simulink model "MRAC_quadrotor_attitude_control"  (R2017a)
settings: Solver=ode45  StartTime=0.0  StopTime=500  FixedStep=0.0001  RelTol=1e3  SampleTimeConstraint=STIndependent  EnableMultiTasking=on
undefined symbols (not defined in the file): DiscIntNeverNeededParam
libraries: dspmtrx3 x6, vrlib x2, neural x1, sharedutil x1
CloseFcn:
  | rtwprivate ssgencode ModelCloseRequest controller
settings Model: Creator=acer  LastModifiedBy=MAQ
settings SolverCC: ZeroCrossControl=DisableAll  AutoInsertRateTranBlk=on
settings DataIOCC: LimitDataPoints=on  SaveFormat=Array  SignalLoggingSaveFormat=ModelDataLogs
settings OptimizationCC: ExpressionDepthLimit=2147483647  LifeSpan=inf
settings DebuggingCC: SaveWithParameterizedLinksMsg=none  UnderspecifiedInitializationDetection=Classic  MergeDetectMultiDrivingBlocksExec=none  SolverPrmCheckMsg=warning  FcnCallInpInsideContextMsg=warning  StateNameClashWarn=warning  SFUnexpectedBacktrackingDiag=warning  SFNoUnconditionalDefaultTransitionDiag=warning  SFExecutionAtInitializationDiag=none
settings HardwareCC: ProdBitPerPointer=32  ProdBitPerSizeT=32  ProdBitPerPtrDiffT=32  ProdLargestAtomicFloat=None  ProdIntDivRoundTo=Undefined  ProdEndianess=Unspecified  ProdWordSize=32  ProdHWDeviceType=32-bit Generic
settings ModelReferenceCC: PropagateSignalLabelsOutOfModel=off
settings GRTTargetCC: TargetLangStandard=C89/C90 (ANSI)  GeneratePreprocessorConditionals=Disable all  CombineOutputUpdateFcns=off  GRTInterface=on
settings ConfigComp: CovMetricSettings=dw  CovHtmlReporting=on  CovSaveCumulativeToWorkspaceVar=on  CovSaveSingleToWorkspaceVar=on  CovExternalEMLEnable=off

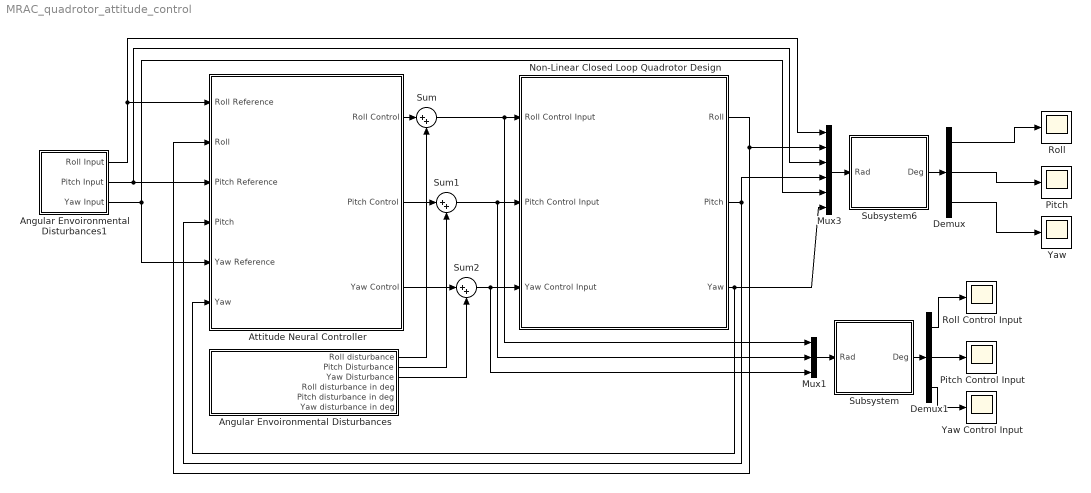
== system MRAC_quadrotor_attitude_control ==
  Angular Envoironmental Disturbances : Subsystem
  Angular Envoironmental Disturbances1 : Subsystem
  Attitude Neural Controller : Subsystem
  Demux : Demux  Outputs=[2,2,2]
  Demux1 : Demux  Outputs=3
  Mux1 : Mux  Inputs=3
  Mux3 : Mux  Inputs=6
  Non-Linear Closed Loop Quadrotor Design : Subsystem
  Pitch : Scope
  Pitch Control Input : Scope
  Roll : Scope
  Roll Control Input : Scope
  Subsystem : Subsystem
  Subsystem6 : Subsystem
  Sum : Sum  Inputs=|++
  Sum1 : Sum  Inputs=|++
  Sum2 : Sum  Inputs=|++
  Yaw : Scope
  Yaw Control Input : Scope
  wires:
  Non-Linear Closed Loop Quadrotor Design/1(Roll) -> Mux3/2, Attitude Neural Controller/2(Roll)
  Angular Envoironmental Disturbances1/1(Roll Input) -> Attitude Neural Controller/1(Roll Reference), Mux3/1
  Demux1/1 -> Roll Control Input/1
  Angular Envoironmental Disturbances1/2(Pitch Input) -> Mux3/3, Attitude Neural Controller/3(Pitch Reference)
  Non-Linear Closed Loop Quadrotor Design/2(Pitch) -> Attitude Neural Controller/4(Pitch), Mux3/4
  Demux1/2 -> Pitch Control Input/1
  Sum1/1 -> Mux1/2, Non-Linear Closed Loop Quadrotor Design/2(Pitch Control Input)
  Sum/1 -> Mux1/1, Non-Linear Closed Loop Quadrotor Design/1(Roll Control Input)
  Sum2/1 -> Mux1/3, Non-Linear Closed Loop Quadrotor Design/3(Yaw Control Input)
  Non-Linear Closed Loop Quadrotor Design/3(Yaw) -> Attitude Neural Controller/6(Yaw), Mux3/6
  Angular Envoironmental Disturbances1/3(Yaw Input) -> Attitude Neural Controller/5(Yaw Reference), Mux3/5
  Demux1/3 -> Yaw Control Input/1
  Mux3/1 -> Subsystem6/1(Rad)
  Subsystem6/1(Deg) -> Demux/1
  Demux/2 -> Pitch/1
  Mux1/1 -> Subsystem/1(Rad)
  Subsystem/1(Deg) -> Demux1/1
  Attitude Neural Controller/3(Yaw Control) -> Sum2/1
  Angular Envoironmental Disturbances/3(Yaw Disturbance) -> Sum2/2
  Attitude Neural Controller/2(Pitch Control) -> Sum1/1
  Angular Envoironmental Disturbances/2(Pitch Disturbance) -> Sum1/2
  Attitude Neural Controller/1(Roll Control) -> Sum/1
  Angular Envoironmental Disturbances/1(Roll disturbance) -> Sum/2
  Demux/1 -> Roll/1
  Demux/3 -> Yaw/1

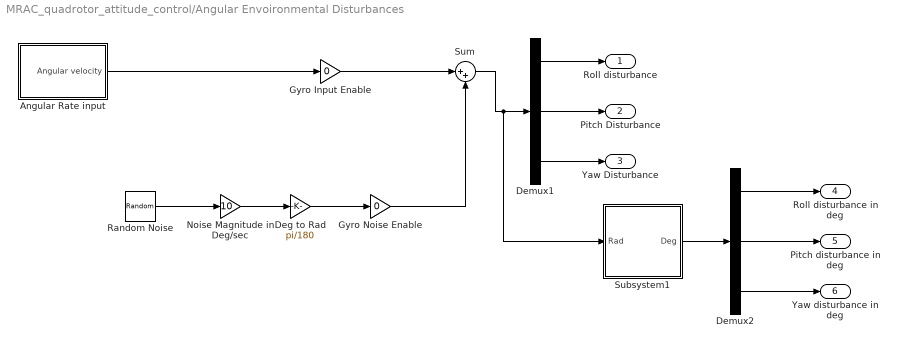
== system MRAC_quadrotor_attitude_control/Angular Envoironmental Disturbances ==
  Angular Rate input : Subsystem
  Deg to Rad : Gain  Gain=pi/180
  Demux1 : Demux  Outputs=3
  Demux2 : Demux  Outputs=3
  Gyro Input Enable : Gain  Gain=0
  Gyro Noise Enable : Gain  Gain=0
  Noise Magnitude in Deg/sec : Gain  Gain=10
  Random Noise : RandomNumber  Variance=0.25  SampleTime=0
  Subsystem1 : Subsystem
  Sum : Sum  Inputs=|++
  Roll disturbance : Outport
  Pitch Disturbance : Outport  Port=2
  Yaw Disturbance : Outport  Port=3
  Roll disturbance in deg : Outport  Port=4
  Pitch disturbance in deg : Outport  Port=5
  Yaw disturbance in deg : Outport  Port=6
  wires:
  Random Noise/1 -> Noise Magnitude in Deg/sec/1
  Sum/1 -> Subsystem1/1(Rad), Demux1/1
  Gyro Noise Enable/1 -> Sum/2
  Angular Rate input/1(Angular velocity) -> Gyro Input Enable/1
  Deg to Rad/1 -> Gyro Noise Enable/1
  Noise Magnitude in Deg/sec/1 -> Deg to Rad/1
  Gyro Input Enable/1 -> Sum/1
  Demux1/1 -> Roll disturbance/1
  Demux1/2 -> Pitch Disturbance/1
  Demux1/3 -> Yaw Disturbance/1
  Subsystem1/1(Deg) -> Demux2/1
  Demux2/1 -> Roll disturbance in deg/1
  Demux2/3 -> Yaw disturbance in deg/1
  Demux2/2 -> Pitch disturbance in deg/1

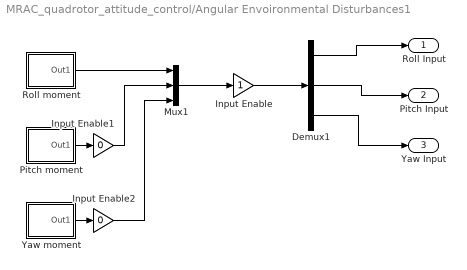
== system MRAC_quadrotor_attitude_control/Angular Envoironmental Disturbances1 ==
  Demux1 : Demux  Outputs=3
  Input Enable : Gain
  Input Enable1 : Gain  Gain=0
  Input Enable2 : Gain  Gain=0
  Mux1 : Mux  Inputs=3
  Pitch moment : Subsystem  mask(timed input){t=[0 100 100 500], u=[0 0 25 25]*pi/180}
      mask prompts: t "time values:"; u "input values"
      mask Display: plot(t,u)
  Roll moment : Subsystem  mask(timed input){t=[0 200 200 500], u=[0 0 20 20]*pi/180}
      mask prompts: t "time values:"; u "input values"
      mask Display: plot(t,u)
  Yaw moment : Subsystem  mask(timed input){t=[0 300 300 500], u=[0 0 10 10]*pi/180}
      mask prompts: t "time values:"; u "input values"
      mask Display: plot(t,u)
  Roll Input : Outport
  Pitch Input : Outport  Port=2
  Yaw Input : Outport  Port=3
  wires:
  Roll moment/1(Out1) -> Mux1/1
  Pitch moment/1(Out1) -> Input Enable1/1
  Yaw moment/1(Out1) -> Input Enable2/1
  Demux1/1 -> Roll Input/1
  Demux1/2 -> Pitch Input/1
  Demux1/3 -> Yaw Input/1
  Input Enable/1 -> Demux1/1
  Mux1/1 -> Input Enable/1
  Input Enable1/1 -> Mux1/2
  Input Enable2/1 -> Mux1/3

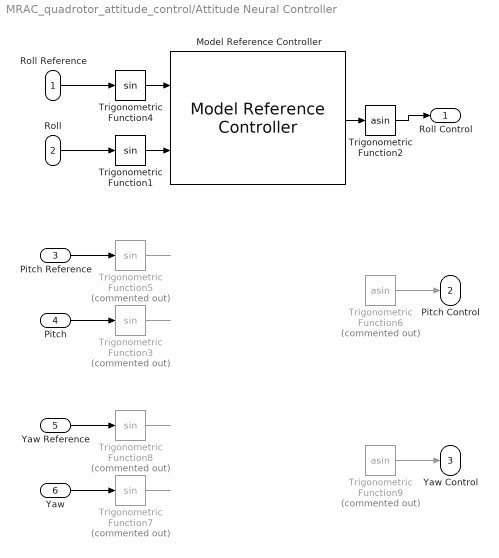
== system MRAC_quadrotor_attitude_control/Attitude Neural Controller ==
  Roll Reference : Inport
  Roll : Inport  Port=2
  Pitch Reference : Inport  Port=3
  Pitch : Inport  Port=4
  Yaw Reference : Inport  Port=5
  Yaw : Inport  Port=6
  Model Reference Controller : neural/Control Systems/Model Reference Controller  Nrc=4  Nic=3  Njc=4  IW_y=[-0.26400634085531088 0.11362328074890946 0.76949015312332025 1.005941348454747;0.36688412438777618 -0.0065967410290466979 -0.72033985218232333 -0.88912388699089739;-0.50358139131277091 0.77939865285332366 0.45366564233329087 0.20305295002900911;0.69691551574309296 0.93834213965429825 0.99228413522118419 0.46539351004482765;-0.59091694955932106 0.27420026736245862 -0.55638905843394881 -0.1844617097356944;-1.1767358237096723 -0.42345585278014547 -1.376668685165205 -1.9008307651836231;0.91466033120602253 -0.41297814120526233 -0.26385222896894323 0.77394756493515449;0.29502607955624394 -0.52311745453581648 -0.39832939881783536 0.37380188688815252;1.0660136206391706 0.91244449330040633 0.99696460523911079 0.49155115383902304;0.63070297319256308 -0.38669531637003984 0.59581348825373337 -0.21032775941831702]  IW_u=[0.56042977945772532 1.0486777442660933 2.1987425118943289;-1.6889164657557667 -0.80321266338753694 -0.9192800619649194;-1.8541863287530997 -0.20017097188284924 -0.60708641279665343;-0.28001378328225929 -1.1150075654652816 1.0207940783869573;-0.70499564957587701 -0.95237632324574006 0.23088874925544114;-0.42189625740733028 -2.3705195154705936 -4.0674084796699121;0.7474100462947203 -1.1953524768000803 -1.3655327562504367;1.3761003380140078 -1.3942056469524908 -0.91047566712262429;1.2032143316328423 1.5376001733686817 0.34323566602274552;-1.1228995990140889 -0.57599779319136679 -1.5199715167734213]  IW_r=[0.13929880088084767 -0.71123019484301042 -0.25515608640194143 -0.041422524854309049;0.13611795317236861 0.019832696517312072 0.70934291910829628 -0.39652942402808944;0.33631471976119631 -0.52824952533632286 -0.60220437280042194 -0.505246106197206;0.30881393403028395 -0.14255401474162388 -0.66488436571113796 0.33691864529663251;0.40040038631379271 1.0480728407462128 0.55697999347242622 -0.030184834439182788;0.90955877692360643 0.95199087143149452 1.0833619369597556 0.34265164308091162;0.67014617449781022 0.61015340408200858 0.74157586751999494 -0.30252864375186672;-0.72603142613625271 -0.12043858389185157 1.0571323958095122 0.37622613209432421;-0.39254518098273627 -1.1001741292886296 0.29052193957884587 -0.33761877898832748;-1.1572293229757462 -0.018972447365077257 -0.29945439714169159 -0.95018887104406002]  B1_c=[0.64282150723717402;-1.0714314143688932;0.15436795978763335;0.73690626046510621;-0.074033003191508698;0.40729244123106328;0.22841516922084279;0.61431964891831858;0.14949779394883281;1.7263533850660762]  B2_c=0.31484879587640524  LW_c=[0.036083219740493624 -0.017033421322474054 -0.44456589280132919 0.06417024420824434 0.59729580944885596 -0.040970357809656605 0.63106519715641407 -0.78172709286945619 -0.16468842249372001 0.060969010733739011]  retraining_c=25  max_i_int=0  min_i_int=0  max_r_int=400  min_r_int=100  Ts=0.05  S1=5  Ni=2  Nj=2  sim_file=0  trainfun=trainlm  Use_validation=0  Use_Testing=1  Use_Inc_training=0  Use_previous_weights=1  max_i=1  min_i=-1  max_r=1  min_r=-1  sam_training=0  sam_training_c=5000  epochs=200  epochs_c=30  minp=-0.93969262078590832  maxp=0.93969262078590832  mint=-0.9848038138280788  maxt=0.93969262078590832  Normalize=0  IW=[-0.025013062042015918 0.004136464686980838;-0.97797176081375736 -0.695916466928859;-0.039432618863616486 -0.0038877108883655742;-0.98427976015700624 -0.48483062015731698;-0.001724540600165126 0.0020387649276496118]  LW1_2=[1.8522611518720808 -0.80388200875864657;-1.5185066206607776 0.20172978663592384;0.40524480460798651 -1.2719330598899341;-1.1018603734955705 1.432108945243316;-1.176149127779192 0.62707492245559471]  LW2_1=[0.62787707146920846 0.0018729990102923592 -0.47303644161933917 0.004122445633035327 -1.6196132281773281]  B1=[-1.7854455549452175;0.68675602723942142;0.43375087295602627;-0.21370894191486062;-0.66468364827367854]  B2=-0.15531704723775702  S1c=10  Limit_output=0  min_output=0  max_output=0  Ref_file=0
      settings: SourceProductName=Neural Network Toolbox  SourceProductBaseCode=NN
  Trigonometric Function1 : Trigonometry
  Trigonometric Function2 : Trigonometry  Operator=asin  OutputSignalType=real
  Trigonometric Function{3,5,7..8} (4 alike) : Trigonometry  Commented=on
  Trigonometric Function4 : Trigonometry
  Trigonometric Function6 : Trigonometry  Commented=on  Operator=asin  OutputSignalType=real
  Trigonometric Function9 : Trigonometry  Commented=on  Operator=asin  OutputSignalType=real
  Roll Control : Outport
  Pitch Control : Outport  Port=2
  Yaw Control : Outport  Port=3
  wires:
  Trigonometric Function5/1 -> ?
  Model Reference Controller/1 -> Trigonometric Function2/1
  Trigonometric Function1/1 -> Model Reference Controller/2
  Trigonometric Function4/1 -> Model Reference Controller/1
  Trigonometric Function3/1 -> ?
  Trigonometric Function6/1 -> Pitch Control/1
  Trigonometric Function2/1 -> Roll Control/1
  ? -> Trigonometric Function6/1
  Pitch/1 -> Trigonometric Function3/1
  Pitch Reference/1 -> Trigonometric Function5/1
  Roll Reference/1 -> Trigonometric Function4/1
  Roll/1 -> Trigonometric Function1/1
  Yaw/1 -> Trigonometric Function7/1
  Yaw Reference/1 -> Trigonometric Function8/1
  ? -> Trigonometric Function9/1
  Trigonometric Function7/1 -> ?
  Trigonometric Function8/1 -> ?
  Trigonometric Function9/1 -> Yaw Control/1

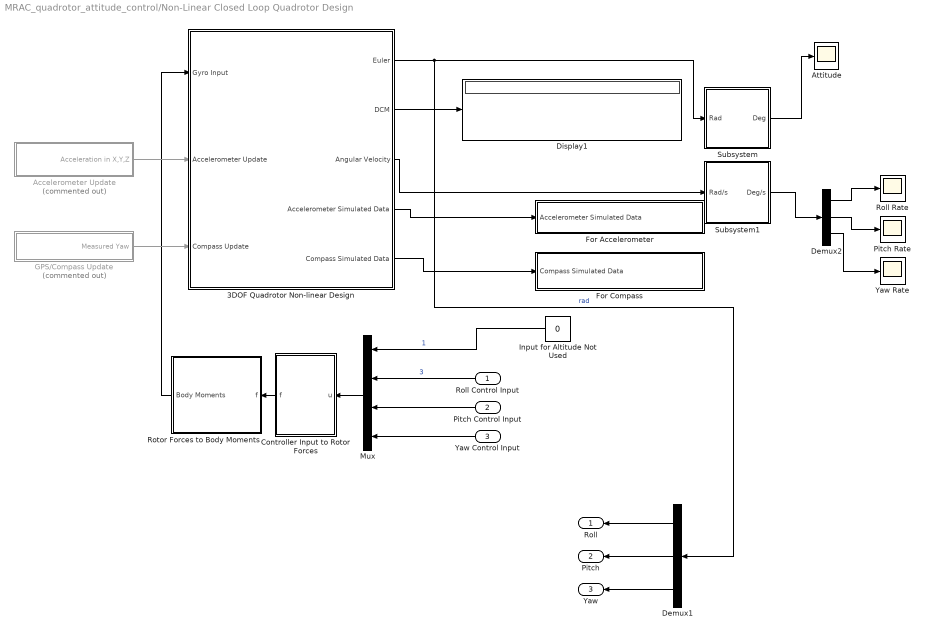
== system MRAC_quadrotor_attitude_control/Non-Linear Closed Loop Quadrotor Design ==
  Roll Control Input : Inport
  Pitch Control Input : Inport  Port=2
  Yaw Control Input : Inport  Port=3
  3DOF Quadrotor Non-linear Design : Subsystem
  Accelerometer Update : Subsystem  Commented=on
  Attitude : Scope
  Controller Input to Rotor Forces : Subsystem
  Demux1 : Demux  Outputs=3
  Demux2 : Demux  Outputs=3
  Display1 : Display
  For Accelerometer : Subsystem
  For Compass : Subsystem
  GPS/Compass Update : Subsystem  Commented=on
  Input for Altitude Not Used : Constant  Value=0
  Mux : Mux
  Pitch Rate : Scope
  Roll Rate : Scope
  Rotor Forces to Body Moments : Subsystem
  Subsystem : Subsystem
  Subsystem1 : Subsystem
  Yaw Rate : Scope
  Roll : Outport
  Pitch : Outport  Port=2
  Yaw : Outport  Port=3
  wires:
  Controller Input to Rotor Forces/1(f) -> Rotor Forces to Body Moments/1(f)
  3DOF Quadrotor Non-linear Design/1(Euler) -> Demux1/1, Subsystem/1(Rad)  "rad"
  Rotor Forces to Body Moments/1(Body Moments) -> 3DOF Quadrotor Non-linear Design/1(Gyro Input)
  Accelerometer Update/1(Acceleration in X,Y,Z) -> 3DOF Quadrotor Non-linear Design/2(Accelerometer Update)
  GPS/Compass Update/1(Measured Yaw) -> 3DOF Quadrotor Non-linear Design/3(Compass Update)
  3DOF Quadrotor Non-linear Design/2(DCM) -> Display1/1
  Subsystem/1(Deg) -> Attitude/1
  Subsystem1/1(Deg/s) -> Demux2/1
  Demux2/1 -> Roll Rate/1
  Demux2/2 -> Pitch Rate/1
  Demux2/3 -> Yaw Rate/1
  3DOF Quadrotor Non-linear Design/3("Angular Velocity ") -> Subsystem1/1(Rad/s)
  3DOF Quadrotor Non-linear Design/4(Accelerometer Simulated Data) -> For Accelerometer/1(Accelerometer Simulated Data)
  3DOF Quadrotor Non-linear Design/5(Compass Simulated Data) -> For Compass/1(Compass Simulated Data)
  Input for Altitude Not Used/1 -> Mux/1  "1"
  Roll Control Input/1 -> Mux/2  "3"
  Mux/1 -> Controller Input to Rotor Forces/1(u)
  Demux1/1 -> Roll/1
  Pitch Control Input/1 -> Mux/3
  Demux1/2 -> Pitch/1
  Yaw Control Input/1 -> Mux/4
  Demux1/3 -> Yaw/1

== system MRAC_quadrotor_attitude_control/Subsystem ==
  Rad : Inport
  Constant : Constant  Value=180/pi
  Product1 : Product  RndMeth=Zero
  Deg : Outport
  wires:
  Constant/1 -> Product1/2
  Rad/1 -> Product1/1
  Product1/1 -> Deg/1

== system MRAC_quadrotor_attitude_control/Subsystem6 ==
  Rad : Inport
  Constant : Constant  Value=180/pi
  Product1 : Product  RndMeth=Zero
  Deg : Outport
  wires:
  Constant/1 -> Product1/2
  Rad/1 -> Product1/1
  Product1/1 -> Deg/1

== system MRAC_quadrotor_attitude_control/Angular Envoironmental Disturbances/Angular Rate input ==
  Mux : Mux  Inputs=3
  Pitch moment : Subsystem  mask(timed input){t=[0 100 100 200 200 300 300 400 400 500], u=[0 0 50 50 0 0 -50 -50 0 0]*pi/180*0}
      mask prompts: t "time values:"; u "input values"
      mask Display: plot(t,u)
  Roll moment : Subsystem  mask(timed input){t=[0 100 100 200 200 300 300 400 400 500], u=[0 0 50 50 0 0 -50 -50 0 0]*pi/180}
      mask prompts: t "time values:"; u "input values"
      mask Display: plot(t,u)
  Yaw moment : Subsystem  mask(timed input){t=[0 200 200 300 300 400 400 500], u=[0 0 45 45 0 0 -45 -45]*pi/180*0}
      mask prompts: t "time values:"; u "input values"
      mask Display: plot(t,u)
  Angular velocity : Outport
  wires:
  Roll moment/1(Out1) -> Mux/1
  Pitch moment/1(Out1) -> Mux/2
  Yaw moment/1(Out1) -> Mux/3
  Mux/1 -> Angular velocity/1

== system MRAC_quadrotor_attitude_control/Angular Envoironmental Disturbances/Subsystem1 ==
  Rad : Inport
  Constant : Constant  Value=180/pi
  Product1 : Product  RndMeth=Zero
  Deg : Outport
  wires:
  Constant/1 -> Product1/2
  Rad/1 -> Product1/1
  Product1/1 -> Deg/1

== system MRAC_quadrotor_attitude_control/Angular Envoironmental Disturbances1/Pitch moment ==
  From Workspace : FromWorkspace  VariableName=[t',u']  SampleTime=0
  Out1 : Outport
  wires:
  From Workspace/1 -> Out1/1

== system MRAC_quadrotor_attitude_control/Angular Envoironmental Disturbances1/Roll moment ==
  From Workspace : FromWorkspace  VariableName=[t',u']  SampleTime=0
  Out1 : Outport
  wires:
  From Workspace/1 -> Out1/1

== system MRAC_quadrotor_attitude_control/Angular Envoironmental Disturbances1/Yaw moment ==
  From Workspace : FromWorkspace  VariableName=[t',u']  SampleTime=0
  Out1 : Outport
  wires:
  From Workspace/1 -> Out1/1

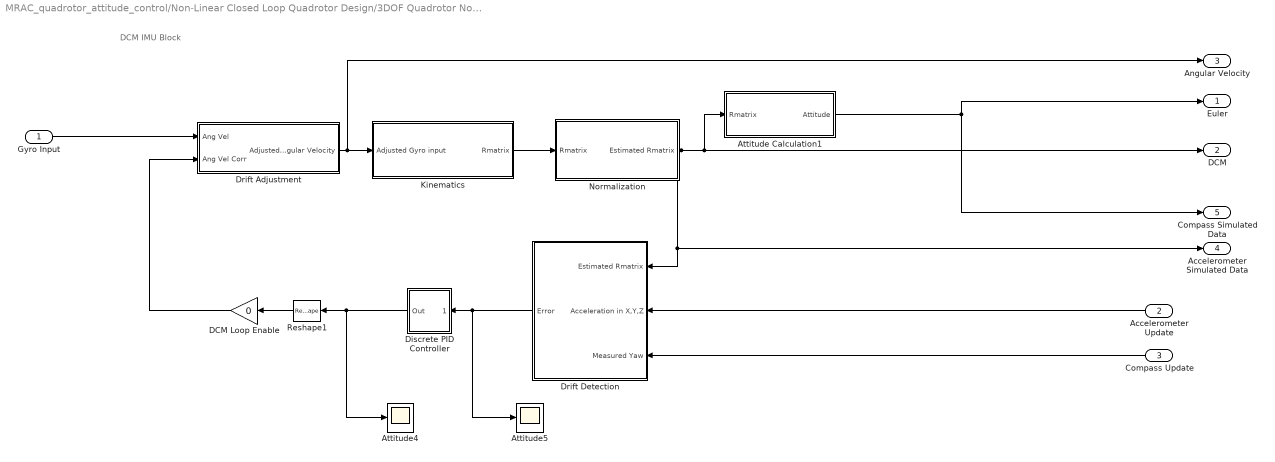
== system MRAC_quadrotor_attitude_control/Non-Linear Closed Loop Quadrotor Design/3DOF Quadrotor Non-linear Design ==
  note: DCM IMU Block
  Gyro Input : Inport
  Accelerometer Update : Inport  Port=2
  Compass Update : Inport  Port=3
  Attitude Calculation1 : Subsystem
  Attitude4 : Scope
  Attitude5 : Scope
  DCM Loop Enable : Gain  Gain=0
  Discrete PID Controller : Subsystem  AncestorBlock=|  DialogController=POWERSYS.PowerSysDialog  mask(Discrete PID Controller){Kp=5, Ki=2, Kd=0, TcD=0, Par_Limits=[1e6 -1e6], Init=0, Ts=1}
      | powerlib_extras/Discrete 
      | Control Blocks/Discrete
      | PID Controller
      mask prompts: Kp "Proportional gain (Kp):"; Ki "Integral gain (Ki):"; Kd "Derivative gain (Kd):"; TcD "Time constant for derivative (s):"; Par_Limits "Output limits: [ Upper   Lower ]"; Init "Output initial value:"; Ts "Sample time:"
      mask help: This block implements a discrete PID controller.
      mask init:
      | UpperLimit=Par_Limits(1);
      | LowerLimit=Par_Limits(2);
      | power_initmask();
      mask Help: This block is part of a subset of blocks in the Extras library that does not have documentation associated with it, other than the block mask description.
      mask Display: disp('PID');
  Drift Adjustment : Subsystem
  Drift Detection : Subsystem
  Kinematics : Subsystem
  Normalization : Subsystem
  Reshape1 : Reshape  OutputDimensionality=Column vector (2-D)
  Euler : Outport
  DCM : Outport  Port=2
  "Angular Velocity " : Outport  Port=3
  Accelerometer Simulated Data : Outport  Port=4
  Compass Simulated Data : Outport  Port=5
  wires:
  Attitude Calculation1/1(Attitude) -> Euler/1, Compass Simulated Data/1
  Drift Adjustment/1(Adjusted Angular Velocity) -> "Angular Velocity "/1, Kinematics/1(Adjusted Gyro input)
  Gyro Input/1 -> Drift Adjustment/1(Ang Vel)
  Compass Update/1 -> Drift Detection/3(Measured Yaw)
  Drift Detection/1(Error) -> Attitude5/1, Discrete PID Controller/1(Error)
  Discrete PID Controller/1(Out) -> Attitude4/1, Reshape1/1
  Accelerometer Update/1 -> Drift Detection/2(Acceleration in X,Y,Z)
  Reshape1/1 -> DCM Loop Enable/1
  DCM Loop Enable/1 -> Drift Adjustment/2(Ang Vel Corr)
  Normalization/1(Estimated Rmatrix) -> Accelerometer Simulated Data/1, Drift Detection/1(Estimated Rmatrix), Attitude Calculation1/1(Rmatrix), DCM/1
  Kinematics/1(Rmatrix) -> Normalization/1(Rmatrix)

== system MRAC_quadrotor_attitude_control/Non-Linear Closed Loop Quadrotor Design/Accelerometer Update ==
  Attitude2 : Scope
  From File : FromFile  FileName=acceleration_from_simulink  SampleTime=0
  Acceleration in X,Y,Z : Outport
  wires:
  From File/1 -> Attitude2/1, Acceleration in X,Y,Z/1

== system MRAC_quadrotor_attitude_control/Non-Linear Closed Loop Quadrotor Design/Controller Input to Rotor Forces ==
  u : Inport
  Matrix Multiply : Product  Multiplication=Matrix(*)
  inv(plant_model) : Constant  Value=|  VectorParams1D=off
      | [  -0.2500         0   -0.5000   -0.2500
      |  ;  -0.2500   -0.5000         0    0.2500
      |   ; -0.2500         0    0.5000   -0.2500
      |   ; -0.2500    0.5000         0    0.2500
      | ]
  f : Outport
  wires:
  inv(plant_model)/1 -> Matrix Multiply/1
  Matrix Multiply/1 -> f/1
  u/1 -> Matrix Multiply/2

== system MRAC_quadrotor_attitude_control/Non-Linear Closed Loop Quadrotor Design/For Accelerometer ==
  Accelerometer Simulated Data : Inport
  Embedded MATLAB Function1 : MATLAB Function  TreatAsAtomicUnit=on
  For acceleration : ToFile  Filename=acceleration_from_simulink.mat
  Mux : Mux  Inputs=3
  wires:
  Embedded MATLAB Function1/1(accel_x) -> Mux/1
  Embedded MATLAB Function1/3(accel_z) -> Mux/3
  Mux/1 -> For acceleration/1
  Embedded MATLAB Function1/2(accel_y) -> Mux/2
  Accelerometer Simulated Data/1 -> Embedded MATLAB Function1/1(R_t_n)

== system MRAC_quadrotor_attitude_control/Non-Linear Closed Loop Quadrotor Design/For Compass ==
  Compass Simulated Data : Inport
  Demux1 : Demux  Outputs=3
  For Compass : ToFile  Filename=yaw_from_simulink
  Terminator1 : Terminator
  Terminator2 : Terminator
  wires:
  Compass Simulated Data/1 -> Demux1/1
  Demux1/2 -> Terminator2/1
  Demux1/1 -> Terminator1/1
  Demux1/3 -> For Compass/1

== system MRAC_quadrotor_attitude_control/Non-Linear Closed Loop Quadrotor Design/GPS//Compass Update ==
  Attitude3 : Scope
  GPS/Compass Update : FromFile  FileName=yaw_from_simulink  SampleTime=0
  Subsystem2 : Subsystem
  Measured Yaw : Outport
  wires:
  GPS/Compass Update/1 -> Subsystem2/1(Rad), Measured Yaw/1
  Subsystem2/1(Deg) -> Attitude3/1

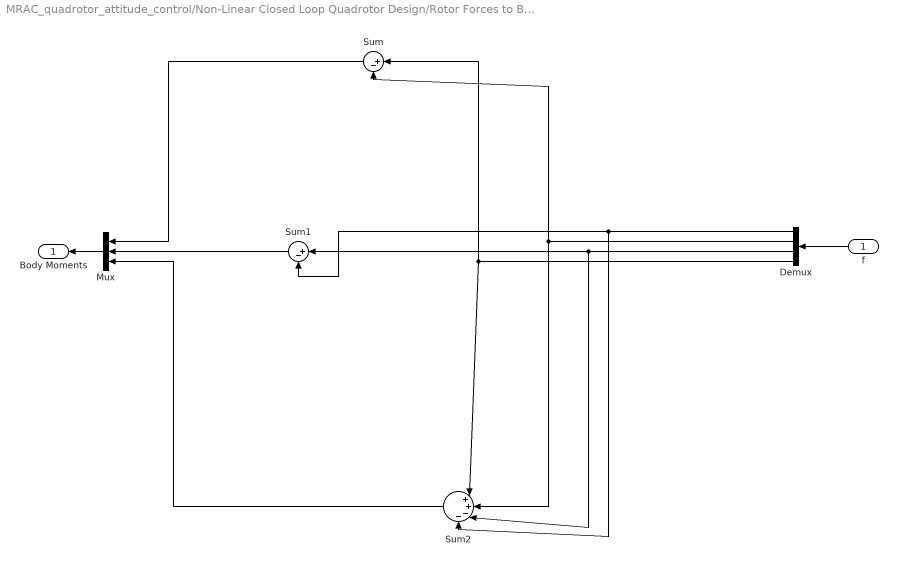
== system MRAC_quadrotor_attitude_control/Non-Linear Closed Loop Quadrotor Design/Rotor Forces to Body Moments ==
  f : Inport
  Demux : Demux
  Mux : Mux  Inputs=3
  Sum : Sum  Inputs=|+-
  Sum1 : Sum  Inputs=|+-
  Sum2 : Sum  Inputs=|++--
  Body Moments : Outport
  wires:
  Sum/1 -> Mux/1
  Sum1/1 -> Mux/2
  Sum2/1 -> Mux/3
  f/1 -> Demux/1
  Mux/1 -> Body Moments/1
  Demux/1 -> Sum1/2, Sum2/4
  Demux/2 -> Sum2/2, Sum/2
  Demux/3 -> Sum1/1, Sum2/3
  Demux/4 -> Sum2/1, Sum/1

== system MRAC_quadrotor_attitude_control/Non-Linear Closed Loop Quadrotor Design/Subsystem ==
  Rad : Inport
  Constant : Constant  Value=180/pi
  Product1 : Product  RndMeth=Zero
  Deg : Outport
  wires:
  Constant/1 -> Product1/2
  Rad/1 -> Product1/1
  Product1/1 -> Deg/1

== system MRAC_quadrotor_attitude_control/Non-Linear Closed Loop Quadrotor Design/Subsystem1 ==
  Rad/s : Inport
  Constant : Constant  Value=180/pi
  Product1 : Product  RndMeth=Zero
  Deg/s : Outport
  wires:
  Constant/1 -> Product1/2
  Rad/s/1 -> Product1/1
  Product1/1 -> Deg/s/1

== system MRAC_quadrotor_attitude_control/Angular Envoironmental Disturbances/Angular Rate input/Pitch moment ==
  From Workspace : FromWorkspace  VariableName=[t',u']  SampleTime=0
  Out1 : Outport
  wires:
  From Workspace/1 -> Out1/1

== system MRAC_quadrotor_attitude_control/Angular Envoironmental Disturbances/Angular Rate input/Roll moment ==
  From Workspace : FromWorkspace  VariableName=[t',u']  SampleTime=0
  Out1 : Outport
  wires:
  From Workspace/1 -> Out1/1

== system MRAC_quadrotor_attitude_control/Angular Envoironmental Disturbances/Angular Rate input/Yaw moment ==
  From Workspace : FromWorkspace  VariableName=[t',u']  SampleTime=0
  Out1 : Outport
  wires:
  From Workspace/1 -> Out1/1

== system MRAC_quadrotor_attitude_control/Non-Linear Closed Loop Quadrotor Design/3DOF Quadrotor Non-linear Design/Attitude Calculation1 ==
  Rmatrix : Inport
  Embedded MATLAB Function1 : MATLAB Function  TreatAsAtomicUnit=on
  Mux : Mux  Inputs=3
  Attitude : Outport
  wires:
  Embedded MATLAB Function1/1(Roll) -> Mux/1
  Mux/1 -> Attitude/1
  Rmatrix/1 -> Embedded MATLAB Function1/1(R_mat)
  Embedded MATLAB Function1/2(Pitch) -> Mux/2
  Embedded MATLAB Function1/3(Yaw) -> Mux/3

== system MRAC_quadrotor_attitude_control/Non-Linear Closed Loop Quadrotor Design/3DOF Quadrotor Non-linear Design/Discrete PID Controller ==
  note: Pierre Giroux, Gilbert Sybille
      | Power System Simulation Laboratory
      | IREQ, Hydro-Quebc
  note: Discrete PID Controller
  Error : Inport
  Discrete-Time Integrator : DiscreteIntegrator  InitialCondition=Init  SampleTime=Ts  LimitOutput=on  UpperSaturationLimit=UpperLimit  LowerSaturationLimit=LowerLimit  ICPrevOutput=DiscIntNeverNeededParam  ICPrevScaledInput=DiscIntNeverNeededParam
  Kp4 : Gain  Gain=Kp  SaturateOnIntegerOverflow=on  OutDataTypeStr=Inherit: Same as input  ParamDataTypeStr=Inherit: Same as input
  Kp5 : Gain  Gain=Ki  SaturateOnIntegerOverflow=on  OutDataTypeStr=Inherit: Same as input  ParamDataTypeStr=Inherit: Same as input
  Saturation2 : Saturate  UpperLimit=UpperLimit  LowerLimit=LowerLimit
  Sum6 : Sum  SaturateOnIntegerOverflow=on  InputSameDT=on  OutDataTypeStr=Inherit: Same as first input
  Out : Outport  InitialOutput=0
  wires:
  Error/1 -> Kp4/1, Kp5/1
  Sum6/1 -> Saturation2/1
  Kp5/1 -> Discrete-Time Integrator/1
  Kp4/1 -> Sum6/1
  Discrete-Time Integrator/1 -> Sum6/2
  Saturation2/1 -> Out/1

== system MRAC_quadrotor_attitude_control/Non-Linear Closed Loop Quadrotor Design/3DOF Quadrotor Non-linear Design/Drift Adjustment ==
  Ang Vel : Inport
  Ang Vel Corr : Inport  Port=2
  Sum : Sum  Inputs=|+-
  Adjusted Angular Velocity : Outport
  wires:
  Ang Vel/1 -> Sum/1
  Sum/1 -> Adjusted Angular Velocity/1
  Ang Vel Corr/1 -> Sum/2

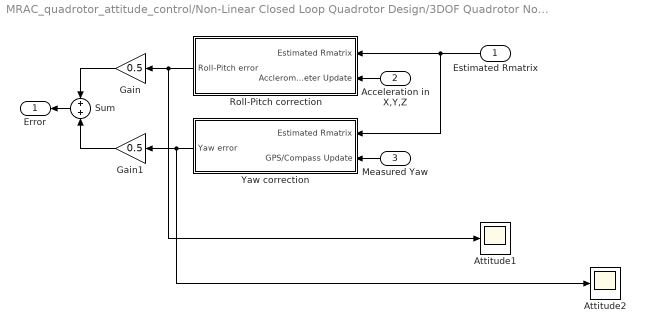
== system MRAC_quadrotor_attitude_control/Non-Linear Closed Loop Quadrotor Design/3DOF Quadrotor Non-linear Design/Drift Detection ==
  Estimated Rmatrix : Inport
  Acceleration in X,Y,Z : Inport  Port=2
  Measured Yaw : Inport  Port=3
  Attitude1 : Scope
  Attitude2 : Scope
  Gain : Gain  Gain=0.5
  Gain1 : Gain  Gain=0.5
  Roll-Pitch correction : Subsystem
  Sum : Sum
  Yaw correction : Subsystem
  Error : Outport
  wires:
  Roll-Pitch correction/1(Roll-Pitch error) -> Attitude1/1, Gain/1
  Yaw correction/1(Yaw error) -> Attitude2/1, Gain1/1
  Estimated Rmatrix/1 -> Roll-Pitch correction/1(Estimated Rmatrix), Yaw correction/1(Estimated Rmatrix)
  Acceleration in X,Y,Z/1 -> Roll-Pitch correction/2(Acclerometer Update)
  Measured Yaw/1 -> Yaw correction/2(GPS/Compass Update)
  Sum/1 -> Error/1
  Gain/1 -> Sum/1
  Gain1/1 -> Sum/2

== system MRAC_quadrotor_attitude_control/Non-Linear Closed Loop Quadrotor Design/3DOF Quadrotor Non-linear Design/Kinematics ==
  Adjusted Gyro input : Inport
  Demux : Demux  Outputs=3
  Embedded MATLAB Function : MATLAB Function  TreatAsAtomicUnit=on
  Memory : Memory
  Rmatrix : Outport
  wires:
  Demux/1 -> Embedded MATLAB Function/1(R_rate)
  Demux/2 -> Embedded MATLAB Function/2(P_rate)
  Demux/3 -> Embedded MATLAB Function/3(Y_rate)
  Embedded MATLAB Function/1(R_t) -> Memory/1, Rmatrix/1
  Memory/1 -> Embedded MATLAB Function/4(R_t_i)
  Adjusted Gyro input/1 -> Demux/1

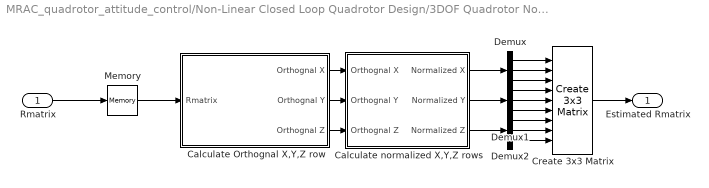
== system MRAC_quadrotor_attitude_control/Non-Linear Closed Loop Quadrotor Design/3DOF Quadrotor Non-linear Design/Normalization ==
  Rmatrix : Inport
  Calculate Orthognal X,Y,Z row : Subsystem
  Calculate normalized X,Y,Z rows : Subsystem
  Create 3x3 Matrix : sharedutil/Create 3x3 Matrix
  Demux : Demux  Outputs=3
  Demux1 : Demux  Outputs=3
  Demux2 : Demux  Outputs=3
  Memory : Memory
  Estimated Rmatrix : Outport
  wires:
  Calculate normalized X,Y,Z rows/1(Normalized X) -> Demux/1
  Calculate normalized X,Y,Z rows/2(Normalized Y) -> Demux1/1
  Calculate normalized X,Y,Z rows/3(Normalized Z) -> Demux2/1
  Demux/1 -> Create 3x3 Matrix/1
  Demux/2 -> Create 3x3 Matrix/2
  Demux/3 -> Create 3x3 Matrix/3
  Demux1/1 -> Create 3x3 Matrix/4
  Demux1/2 -> Create 3x3 Matrix/5
  Demux1/3 -> Create 3x3 Matrix/6
  Demux2/1 -> Create 3x3 Matrix/7
  Demux2/2 -> Create 3x3 Matrix/8
  Demux2/3 -> Create 3x3 Matrix/9
  Calculate Orthognal X,Y,Z row/1(Orthognal X) -> Calculate normalized X,Y,Z rows/1(Orthognal X)
  Calculate Orthognal X,Y,Z row/2(Orthognal Y) -> Calculate normalized X,Y,Z rows/2(Orthognal Y)
  Calculate Orthognal X,Y,Z row/3(Orthognal Z) -> Calculate normalized X,Y,Z rows/3(Orthognal Z)
  Rmatrix/1 -> Memory/1
  Create 3x3 Matrix/1 -> Estimated Rmatrix/1
  Memory/1 -> Calculate Orthognal X,Y,Z row/1(Rmatrix)

== system MRAC_quadrotor_attitude_control/Non-Linear Closed Loop Quadrotor Design/GPS//Compass Update/Subsystem2 ==
  Rad : Inport
  Constant : Constant  Value=180/pi
  Product1 : Product  RndMeth=Zero
  Deg : Outport
  wires:
  Constant/1 -> Product1/2
  Rad/1 -> Product1/1
  Product1/1 -> Deg/1

== system MRAC_quadrotor_attitude_control/Non-Linear Closed Loop Quadrotor Design/3DOF Quadrotor Non-linear Design/Drift Detection/Roll-Pitch correction ==
  Estimated Rmatrix : Inport
  Acclerometer Update : Inport  Port=2
  Cross Product : vrlib/Utilities/Cross Product
      settings: SourceProductBaseCode=VR
  Row 3 selection : dspmtrx3/Submatrix  RowSpan=One row  RowStartMode=Last  RowStartIndex=1  RowEndMode=Last  RowEndIndex=1  ColSpan=All columns  ColStartMode=Last  ColStartIndex=1  ColEndMode=Last  ColEndIndex=1
  Roll-Pitch error : Outport
  wires:
  Estimated Rmatrix/1 -> Row 3 selection/1
  Cross Product/1 -> Roll-Pitch error/1
  Acclerometer Update/1 -> Cross Product/2
  Row 3 selection/1 -> Cross Product/1

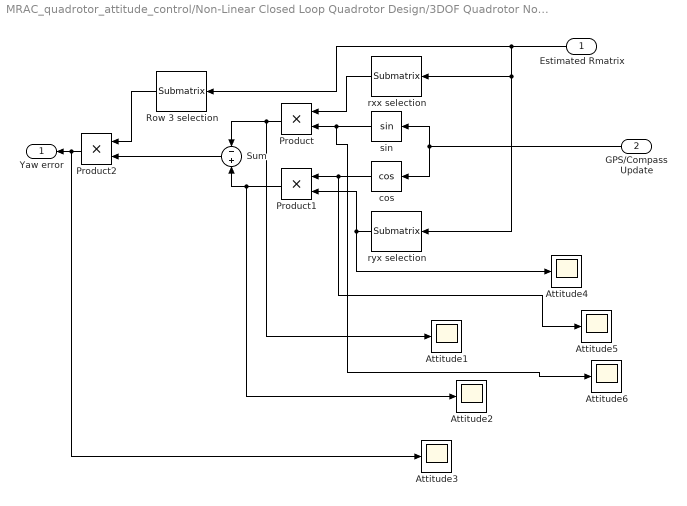
== system MRAC_quadrotor_attitude_control/Non-Linear Closed Loop Quadrotor Design/3DOF Quadrotor Non-linear Design/Drift Detection/Yaw correction ==
  Estimated Rmatrix : Inport
  GPS/Compass Update : Inport  Port=2
  Attitude{1..6} (6 alike) : Scope
  Product : Product  RndMeth=Zero
  Product1 : Product  RndMeth=Zero
  Product2 : Product  RndMeth=Zero
  Row 3 selection : dspmtrx3/Submatrix  RowSpan=One row  RowStartMode=Last  RowStartIndex=1  RowEndMode=Last  RowEndIndex=1  ColSpan=All columns  ColStartMode=First  ColStartIndex=1  ColEndMode=Last  ColEndIndex=1
  Sum : Sum  Inputs=-+
  cos : Trigonometry  Operator=cos
  rxx selection : dspmtrx3/Submatrix  RowSpan=One row  RowStartMode=First  RowStartIndex=1  RowEndMode=Last  RowEndIndex=1  ColSpan=One column  ColStartMode=First  ColStartIndex=1  ColEndMode=Last  ColEndIndex=1
  ryx selection : dspmtrx3/Submatrix  RowSpan=One row  RowStartMode=Middle  RowStartIndex=1  RowEndMode=Last  RowEndIndex=1  ColSpan=One column  ColStartMode=First  ColStartIndex=1  ColEndMode=Last  ColEndIndex=1
  sin : Trigonometry
  Yaw error : Outport
  wires:
  rxx selection/1 -> Product/1
  sin/1 -> Attitude6/1, Product/2
  ryx selection/1 -> Product1/2, Attitude4/1
  cos/1 -> Attitude5/1, Product1/1
  Product/1 -> Attitude1/1, Sum/1
  Product1/1 -> Attitude2/1, Sum/2
  Row 3 selection/1 -> Product2/1
  Sum/1 -> Product2/2
  Estimated Rmatrix/1 -> Row 3 selection/1, ryx selection/1, rxx selection/1
  GPS/Compass Update/1 -> cos/1, sin/1
  Product2/1 -> Attitude3/1, Yaw error/1

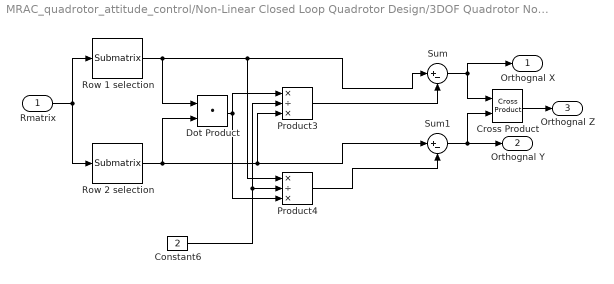
== system MRAC_quadrotor_attitude_control/Non-Linear Closed Loop Quadrotor Design/3DOF Quadrotor Non-linear Design/Normalization/Calculate Orthognal X,Y,Z row ==
  Rmatrix : Inport
  Constant6 : Constant  Value=2
  Cross Product : vrlib/Utilities/Cross Product
      settings: SourceProductBaseCode=VR
  Dot Product : DotProduct  InputSameDT=on  OutDataTypeStr=Inherit: Inherit via internal rule
  Product3 : Product  Inputs=*/*  RndMeth=Zero
  Product4 : Product  Inputs=*/*  RndMeth=Zero
  Row 1 selection : dspmtrx3/Submatrix  RowSpan=One row  RowStartMode=First  RowStartIndex=1  RowEndMode=Last  RowEndIndex=1  ColSpan=All columns  ColStartMode=First  ColStartIndex=1  ColEndMode=Last  ColEndIndex=1
  Row 2 selection : dspmtrx3/Submatrix  RowSpan=One row  RowStartMode=Middle  RowStartIndex=1  RowEndMode=Last  RowEndIndex=1  ColSpan=All columns  ColStartMode=First  ColStartIndex=1  ColEndMode=Last  ColEndIndex=1
  Sum : Sum  Inputs=|+-
  Sum1 : Sum  Inputs=|+-
  Orthognal X : Outport
  Orthognal Y : Outport  Port=2
  Orthognal Z : Outport  Port=3
  wires:
  Sum/1 -> Cross Product/1, Orthognal X/1
  Sum1/1 -> Cross Product/2, Orthognal Y/1
  Row 1 selection/1 -> Product4/1, Sum/1, Dot Product/1
  Row 2 selection/1 -> Product3/3, Sum1/1, Dot Product/2
  Constant6/1 -> Product3/2, Product4/2
  Product3/1 -> Sum/2
  Product4/1 -> Sum1/2
  Cross Product/1 -> Orthognal Z/1
  Rmatrix/1 -> Row 1 selection/1, Row 2 selection/1
  Dot Product/1 -> Product4/3, Product3/1

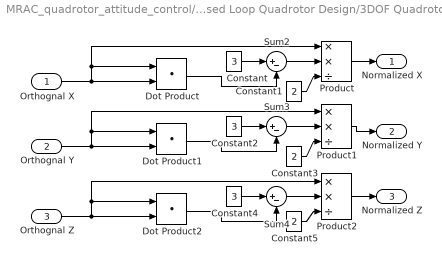
== system MRAC_quadrotor_attitude_control/Non-Linear Closed Loop Quadrotor Design/3DOF Quadrotor Non-linear Design/Normalization/Calculate normalized X,Y,Z rows ==
  Orthognal X : Inport
  Orthognal Y : Inport  Port=2
  Orthognal Z : Inport  Port=3
  Constant : Constant  Value=3
  Constant1 : Constant  Value=2
  Constant2 : Constant  Value=3
  Constant3 : Constant  Value=2
  Constant4 : Constant  Value=3
  Constant5 : Constant  Value=2
  Dot Product : DotProduct  InputSameDT=on  OutDataTypeStr=Inherit: Inherit via internal rule
  Dot Product1 : DotProduct  InputSameDT=on  OutDataTypeStr=Inherit: Inherit via internal rule
  Dot Product2 : DotProduct  InputSameDT=on  OutDataTypeStr=Inherit: Inherit via internal rule
  Product : Product  Inputs=**/  RndMeth=Zero
  Product1 : Product  Inputs=**/  RndMeth=Zero
  Product2 : Product  Inputs=**/  RndMeth=Zero
  Sum2 : Sum  Inputs=|+-
  Sum3 : Sum  Inputs=|+-
  Sum4 : Sum  Inputs=|+-
  Normalized X : Outport
  Normalized Y : Outport  Port=2
  Normalized Z : Outport  Port=3
  wires:
  Constant/1 -> Sum2/1
  Sum2/1 -> Product/2
  Constant1/1 -> Product/3
  Constant2/1 -> Sum3/1
  Sum3/1 -> Product1/2
  Constant3/1 -> Product1/3
  Constant4/1 -> Sum4/1
  Sum4/1 -> Product2/2
  Constant5/1 -> Product2/3
  Product/1 -> Normalized X/1
  Product1/1 -> Normalized Y/1
  Product2/1 -> Normalized Z/1
  Orthognal X/1 -> Dot Product/2, Dot Product/1, Product/1
  Dot Product/1 -> Sum2/2
  Orthognal Y/1 -> Dot Product1/2, Dot Product1/1, Product1/1
  Dot Product1/1 -> Sum3/2
  Orthognal Z/1 -> Dot Product2/2, Dot Product2/1, Product2/1
  Dot Product2/1 -> Sum4/2

== matlab function MRAC_quadrotor_attitude_control/Non-Linear Closed Loop Quadrotor Design/3DOF Quadrotor Non-linear Design/Kinematics/Embedded MATLAB Function ==
  data: R_rate input; R_t output; P_rate input; Y_rate input; R_t_i input
function R_t= fcn(R_rate,P_rate,Y_rate,R_t_i)
%--------------------Calculate Change in Rmatrix-------------------
dt=0.01;
a11=1;
a22=1;
a33=1;
a12=-Y_rate*dt;
a13=P_rate*dt;
a21=Y_rate*dt;
a23=-R_rate*dt;
a31=-P_rate*dt;
a32=R_rate*dt;
R_dt=[a11 a12 a13;a21 a22 a23;a31 a32 a33];
%--------------------Update Rmatrix-------------------------------
if (det(R_t_i)==0)
    R_t=[1 0 0;0 1 0;0 0 1];
else R_t=R_t_i;
end

R_t=R_t*R_dt;
% R_t=R_dt*R_t;

== matlab function MRAC_quadrotor_attitude_control/Non-Linear Closed Loop Quadrotor Design/For Accelerometer/Embedded MATLAB Function1 ==
  data: R_t_n input; accel_x output; accel_y output; accel_z output
function [accel_x,accel_y,accel_z] = fcn(R_t_n)
Roll = atan2(R_t_n(3,2),R_t_n(3,3));
acc_x=(9.8160*R_t_n(3,1));     %at the moment we are calculating
acc_y=(9.8160*sin(Roll));     %gravity vector in X,Y,Z directions
acc_z=sqrt(9.8160^2-(acc_y)^2-(acc_x)^2);
accel_x=acc_x/sqrt(acc_x^2+acc_y^2+acc_z^2);
accel_y=acc_y/sqrt(acc_x^2+acc_y^2+acc_z^2);
accel_z=acc_z/sqrt(acc_x^2+acc_y^2+acc_z^2);

== matlab function MRAC_quadrotor_attitude_control/Non-Linear Closed Loop Quadrotor Design/3DOF Quadrotor Non-linear Design/Attitude Calculation1/Embedded MATLAB Function1 ==
  data: R_mat input; Roll output; Pitch output; Yaw output
function [Roll, Pitch, Yaw] = asin(R_mat)
% Roll = atan2(u(2,3),u(3,3));
% Pitch=-asin(u(1,3));
% Yaw=atan2(u(1,2),u(1,1));
Roll = atan2(R_mat(3,2),R_mat(3,3));
Pitch=-asin(R_mat(3,1));
Yaw=atan2(R_mat(2,1),R_mat(1,1));
